simulink model "sampleModel83"  (R2021b)
settings: Solver=VariableStepAuto  StartTime=0.0  StopTime=10.0  RelTol=1e-3
libraries: simulink x5, slpidlib x1
settings Model: Creator=user  LastModifiedBy=user

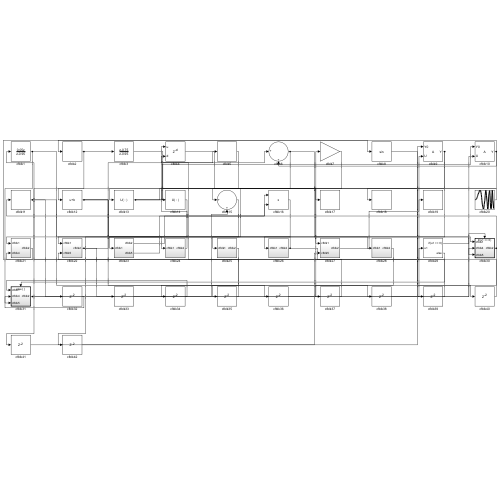
[thumbnail: Simulink's stored preview of the top-level diagram]
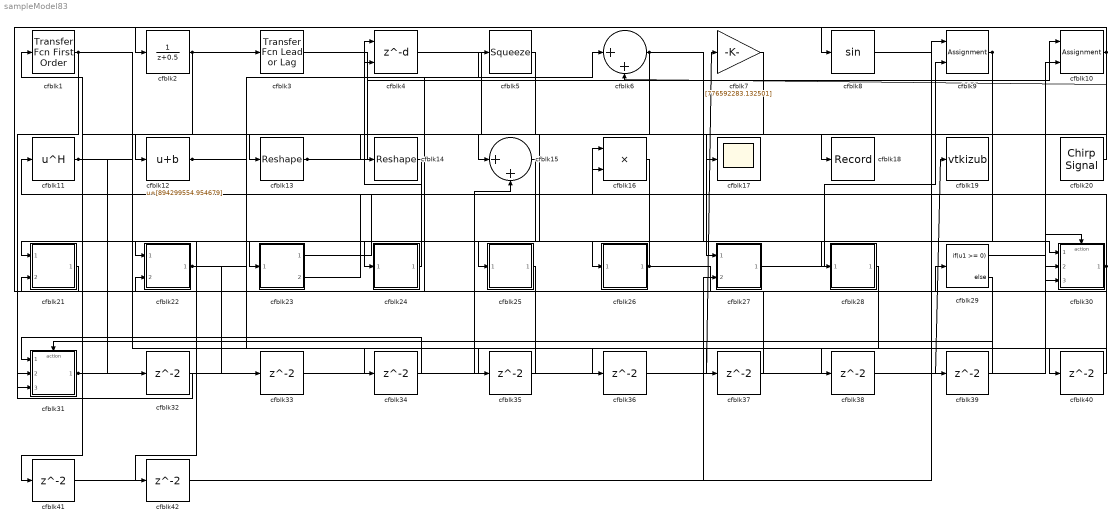
== system sampleModel83 ==
  cfblk1 : simulink/Discrete/Transfer Fcn First Order  PoleZ=0.95  ICPrevOutput=0.0  DoSatur=off
  cfblk10 : Assignment  DiagnosticForDimensions=Warning  IndexOptions=Index vector (dialog)  Indices=1  OutputSizes=1
  cfblk11 : Math  Operator=hermitian  SaturateOnIntegerOverflow=on
  cfblk12 : Bias  Bias=[894299554.954679]
  cfblk13 : Reshape
  cfblk14 : Reshape
  cfblk15 : Sum  Inputs=|++
  cfblk16 : Product  Inputs=**
  cfblk17 : Scope
  cfblk18 : Record  FileSettingsInternal="{\"entries\":[{\"content\":{\"excelSettings\":{\"content\":{},\"type\":\"Streamout.ExcelSettings\"}},\"type\":\"Streamout.FileSettingStorage\",\"uuid\":\"c5e63c93-1856-451a-8116-f2208fe92cf5\"}],\"packageUris\":[\"http://schema.mathworks.com/mf0/streamout_blocks/R2020a\"],\"version\":\"1.0\"}"  SignalsInternal="{\"entries\":[{\"content\":{\"signals\":[{\"content\":{\"blockPath\":[\"sampleModel83/cfblk18\"],\"channel\":[],\"dimensions\":[1],\"domain\":\"sampleModel83/cfblk18\",\"lineColor\":\"#ff13a6\",\"plots\":[1],\"port\":1,\"sid\":[\"\"],\"signalID\":3006,\"signalName\":\"cfblk20\"},\"type\":\"RecordBlkView.Signal\",\"uuid\":\"c2600ee0-9323-4bc2-8a6f-d5c2b001d0d8\"}]},\"type\":\"RecordBlkView.InputSignals\",\"uuid\":\"f8298611-841b-4f7e-947a-f36ca654fdb6\"}],\"packageUris\":[\"http://schema.mathworks.com/mf0/streamout_blocks/R2020a\"],\"version\":\"1.0\"}"  VisualizationBindings="{\"sparklinesplugin\":{\"info\":[{\"bindingParametersList\":[],\"subplotID\":1}]}}"
  cfblk19 : ToWorkspace  VariableName=vtkizub  SaveFormat=Timeseries  SampleTime=-1
  cfblk2 : DiscreteTransferFcn  SampleTime=1
  cfblk20 : simulink/Sources/Chirp Signal  f1=[329950001.186979]  T=[589101481.241266]  f2=[490068830.966682]
  cfblk21 : Subsystem
  cfblk22 : Subsystem
  cfblk23 : Subsystem
  cfblk24 : Subsystem
  cfblk25 : Subsystem
  cfblk26 : Subsystem
  cfblk27 : Subsystem
  cfblk28 : Subsystem
  cfblk29 : If  IfExpression=u1 >= 0  SampleTime=1
  cfblk3 : simulink/Discrete/Transfer Fcn Lead or Lag  PoleZ=0.95  ZeroZ=0.75  ICPrevOutput=0.0  ICPrevInput=0.0  DoSatur=off
      settings: SourceProductBaseCode=SL
  cfblk30 : Subsystem  TreatAsAtomicUnit=on
  cfblk31 : Subsystem  TreatAsAtomicUnit=on
  cfblk{32..42} (11 alike) : Delay  SampleTime=1
  cfblk4 : Delay  DelayLengthSource=Input port  SampleTime=1
      settings: InputPortMap=u0,p1
  cfblk5 : Squeeze
  cfblk6 : Sum  Inputs=|++
  cfblk7 : Gain  Gain=[776592283.132501]
  cfblk8 : Trigonometry
  cfblk9 : Assignment  DiagnosticForDimensions=Warning  IndexOptions=Index vector (dialog)  Indices=1  OutputSizes=1
  wires:
  cfblk15/1 -> cfblk22/1(cfblk1)
  cfblk7/1 -> cfblk15/1
  cfblk26/1(cfblk2) -> cfblk21/1(cfblk1), cfblk29/1
  cfblk2/1 -> cfblk12/1, cfblk3/1
  cfblk20/1 -> cfblk18/1
  cfblk21/1(cfblk2) -> cfblk8/1
  cfblk16/1 -> cfblk26/1(cfblk1)
  cfblk6/1 -> cfblk25/1(cfblk1), cfblk28/1(cfblk1)
  cfblk11/1 -> cfblk32/1, cfblk36/1
  cfblk9/1 -> cfblk13/1, cfblk42/1
  cfblk31/1(cfblk2) -> cfblk7/1, cfblk19/1
  cfblk10/1 -> cfblk2/1, cfblk6/2, cfblk14/1
  cfblk24/1(cfblk2) -> cfblk4/1
  cfblk27/1(cfblk2) -> cfblk9/2
  cfblk4/1 -> cfblk27/1(cfblk1)
  cfblk1/1 -> cfblk24/1(cfblk1), cfblk31/3(cfblk5)
  cfblk14/1 -> cfblk23/1(cfblk1)
  cfblk12/1 -> cfblk30/1(cfblk1), cfblk30/3(cfblk5), cfblk38/1
  cfblk22/1(cfblk2) -> cfblk6/1, cfblk33/1
  cfblk13/1 -> cfblk10/1, cfblk5/1, cfblk17/1
  cfblk23/1(cfblk2) -> cfblk16/1
  cfblk23/2(cfblk5) -> cfblk16/2
  cfblk30/1(cfblk2) -> cfblk11/1, cfblk37/1
  cfblk29/1 -> cfblk30/Action
  cfblk29/2 -> cfblk31/Action
  cfblk32/1 -> cfblk31/2(cfblk4)
  cfblk33/1 -> cfblk15/2
  cfblk25/1(cfblk2) -> cfblk34/1
  cfblk34/1 -> cfblk31/1(cfblk1)
  cfblk28/1(cfblk2) -> cfblk35/1
  cfblk35/1 -> cfblk22/2(cfblk5)
  cfblk36/1 -> cfblk30/2(cfblk4)
  cfblk37/1 -> cfblk1/1
  cfblk38/1 -> cfblk10/2
  cfblk3/1 -> cfblk39/1
  cfblk39/1 -> cfblk4/2
  cfblk8/1 -> cfblk40/1
  cfblk40/1 -> cfblk21/2(cfblk4)
  cfblk5/1 -> cfblk41/1
  cfblk41/1 -> cfblk9/1
  cfblk42/1 -> cfblk27/2(cfblk5)

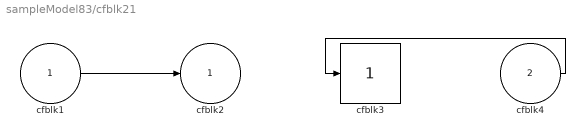
== system sampleModel83/cfblk21 ==
  cfblk1 : Inport
  cfblk4 : Inport  Port=2
  cfblk3 : simulink/Math Operations/Slider Gain  gain=1  low=0  high=2
  cfblk2 : Outport
  wires:
  cfblk4/1 -> cfblk3/1
  cfblk1/1 -> cfblk2/1

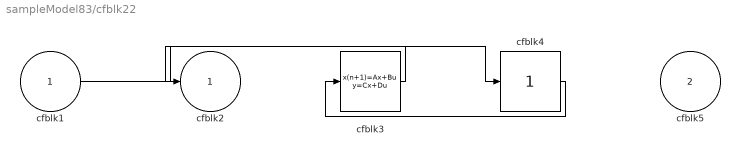
== system sampleModel83/cfblk22 ==
  cfblk1 : Inport
  cfblk5 : Inport  Port=2
  cfblk3 : DiscreteStateSpace
  cfblk4 : simulink/Math Operations/Slider Gain  gain=1  low=0  high=2
  cfblk2 : Outport
  wires:
  cfblk1/1 -> cfblk4/1
  cfblk4/1 -> cfblk3/1
  cfblk3/1 -> cfblk2/1

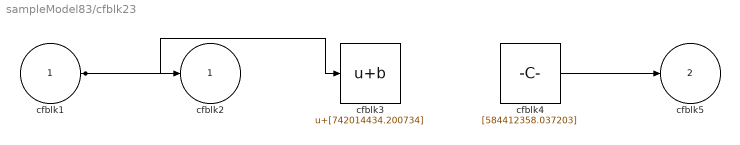
== system sampleModel83/cfblk23 ==
  cfblk1 : Inport
  cfblk3 : Bias  Bias=[742014434.200734]
  cfblk4 : Constant  Value=[584412358.037203]  SampleTime=1
  cfblk2 : Outport
  cfblk5 : Outport  Port=2
  wires:
  cfblk4/1 -> cfblk5/1
  cfblk1/1 -> cfblk2/1, cfblk3/1

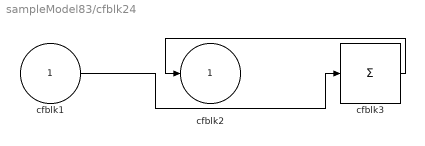
== system sampleModel83/cfblk24 ==
  cfblk1 : Inport
  cfblk3 : Sum  Inputs=+
  cfblk2 : Outport
  wires:
  cfblk3/1 -> cfblk2/1
  cfblk1/1 -> cfblk3/1

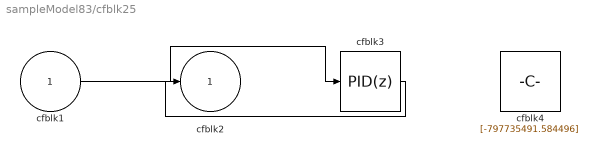
== system sampleModel83/cfblk25 ==
  cfblk1 : Inport
  cfblk3 : slpidlib/PID Controller  Controller=PID  Form=Parallel  TimeDomain=Discrete-time  UseExternalTs=off  SampleTime=1  IntegratorMethod=Forward Euler  FilterMethod=Forward Euler  ControllerParametersSource=internal  P=1  I=1  D=0  UseFilter=on  N=100  TunerSelectOption=Transfer Function Based (PID Tuner App)  InitialConditionSource=internal  InitialConditionForIntegrator=0  InitialConditionForFilter=0  DifferentiatorICPrevScaledInput=0  ExternalReset=none  TrackingMode=off  Kt=1  LimitOutput=off  SatLimitsSource=internal  UpperSaturationLimit=inf  LowerSaturationLimit=-inf  LinearizeAsGain=off  AntiWindupMode=none  Kb=1  POutMin=[]  POutMax=[]  IOutMin=[]  IOutMax=[]  DOutMin=[]  DOutMax=[]  NOutMin=[]  NOutMax=[]  SumOutMin=[]  SumOutMax=[]  SaturationOutMin=[]  SaturationOutMax=[]  PParamMin=[]  PParamMax=[]  IParamMin=[]  IParamMax=[]  DParamMin=[]  DParamMax=[]  NParamMin=[]  NParamMax=[]  KbParamMin=[]  KbParamMax=[]  KtParamMin=[]  KtParamMax=[]  KbOutMin=[]  KbOutMax=[]  KtOutMin=[]  KtOutMax=[]  IntegratorOutMin=[]  IntegratorOutMax=[]  FilterOutMin=[]  FilterOutMax=[]  SumI1OutMin=[]  SumI1OutMax=[]  SumI2OutMin=[]  SumI2OutMax=[]  SumI3OutMin=[]  SumI3OutMax=[]  SumI4OutMin=[]  SumI4OutMax=[]  SumDOutMin=[]  SumDOutMax=[]  DifferentiatorOutMin=[]  DifferentiatorOutMax=[]  FilterDiffOutCoefMin=[]  FilterDiffOutCoefMax=[]  ReciprocalOutMin=[]  ReciprocalOutMax=[]  SumDenOutMin=[]  SumDenOutMax=[]  SumNumOutMin=[]  SumNumOutMax=[]  DivideOutMin=[]  DivideOutMax=[]  UdiffTsProdOutMin=[]  UdiffTsProdOutMax=[]  NTsProdOutMin=[]  NTsProdOutMax=[]  UintegralTsProdOutMin=[]  UintegralTsProdOutMax=[]  UngainTsProdOutMin=[]  UngainTsProdOutMax=[]  IntegratorContinuousStateAttributes=''  IntegratorStateMustResolveToSignalObject=off  IntegratorRTWStateStorageClass=Auto  FilterContinuousStateAttributes=''  FilterStateMustResolveToSignalObject=off  FilterRTWStateStorageClass=Auto  ParallelPVariant=InternalParameters  IdealPVariant=Disabled  IVariant=InternalParameters  DVariant=InternalParameters  IntegratorVariant=Discrete  SatVariant=Disabled  AWVariant=Passthrough  PCopyVariant=Disabled  TRVariant=Disabled  FdbkBlocksVariant=Forward  IdealPFdbkVariant=Disabled  SatFdbkVariant=Disabled  DerivativeFilterVariant=ForwardEulerFilter  NVariant=InternalParameters  NCopyVariant=Disabled  FilterICVariant=InternalICsFilter  IntegratorICVariant=InternalICs  ExternalResetVariant=Disabled  TRSumVariant=Passthrough  SumFdbkVariant=Disabled  SumVariant=Sum_PID  TsampFilterVariant=InternalTs  TsampNgainVariant=Passthrough  TsampIntegralVariant=Passthrough  ExternalSaturationOutDataTypeStr=Inherit: Same as second input
  cfblk4 : Constant  Value=[-797735491.584496]  SampleTime=1
  cfblk2 : Outport
  wires:
  cfblk1/1 -> cfblk3/1
  cfblk3/1 -> cfblk2/1

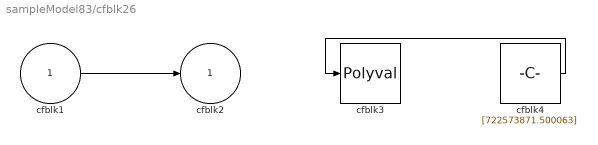
== system sampleModel83/cfblk26 ==
  cfblk1 : Inport
  cfblk3 : Polyval  Coefs=[ +2.081618890e-019, -1.441693666e-014, +4.719686976e-010, -8.536869453e-006, +1.621573104e-001, -8.087801117e+001 ]
  cfblk4 : Constant  Value=[722573871.500063]  SampleTime=1
  cfblk2 : Outport
  wires:
  cfblk4/1 -> cfblk3/1
  cfblk1/1 -> cfblk2/1

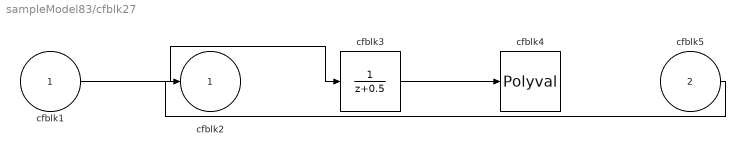
== system sampleModel83/cfblk27 ==
  cfblk1 : Inport
  cfblk5 : Inport  Port=2
  cfblk3 : DiscreteTransferFcn  SampleTime=1
  cfblk4 : Polyval  Coefs=[ +2.081618890e-019, -1.441693666e-014, +4.719686976e-010, -8.536869453e-006, +1.621573104e-001, -8.087801117e+001 ]
  cfblk2 : Outport
  wires:
  cfblk3/1 -> cfblk4/1
  cfblk1/1 -> cfblk3/1
  cfblk5/1 -> cfblk2/1

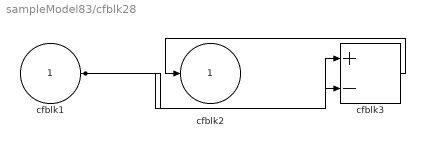
== system sampleModel83/cfblk28 ==
  cfblk1 : Inport
  cfblk3 : Sum  Inputs=+-
  cfblk2 : Outport
  wires:
  cfblk3/1 -> cfblk2/1
  cfblk1/1 -> cfblk3/1, cfblk3/2

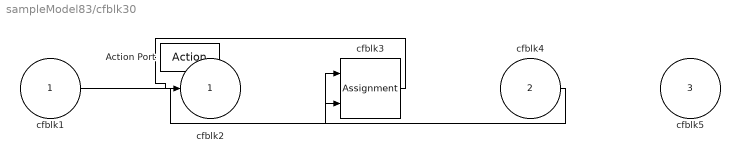
== system sampleModel83/cfblk30 ==
  cfblk1 : Inport
  cfblk4 : Inport  Port=2
  cfblk5 : Inport  Port=3
  Action Port : ActionPort  ActionPortLabel=if(u1 >= 0)
  cfblk3 : Assignment  DiagnosticForDimensions=Warning  IndexOptions=Index vector (dialog)  Indices=1  OutputSizes=1
  cfblk2 : Outport
  wires:
  cfblk1/1 -> cfblk3/1
  cfblk4/1 -> cfblk3/2
  cfblk3/1 -> cfblk2/1

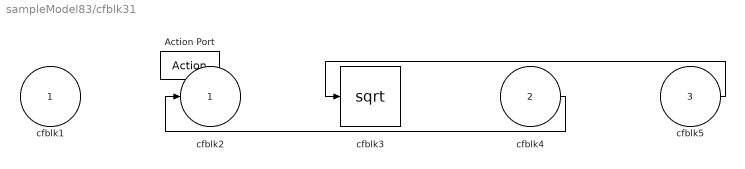
== system sampleModel83/cfblk31 ==
  cfblk1 : Inport
  cfblk4 : Inport  Port=2
  cfblk5 : Inport  Port=3
  Action Port : ActionPort  ActionPortLabel=else
  cfblk3 : Sqrt  SaturateOnIntegerOverflow=on
  cfblk2 : Outport
  wires:
  cfblk4/1 -> cfblk2/1
  cfblk5/1 -> cfblk3/1
